simulink model "ProbeModel_Real"  (R2025a)
settings: Solver=ode23tb  StartTime=0.0  StopTime=1000  MaxStep=0.1  RelTol=1e-3
model workspace (MAT data in the model file):
  probe_base_wl = 88.24
  probe_top_wl = 103.68
libraries: simulink x2
settings Model: DataDictionary=FuelGaugingData.sldd  Creator=mkelley  LastModifiedBy=mkelley

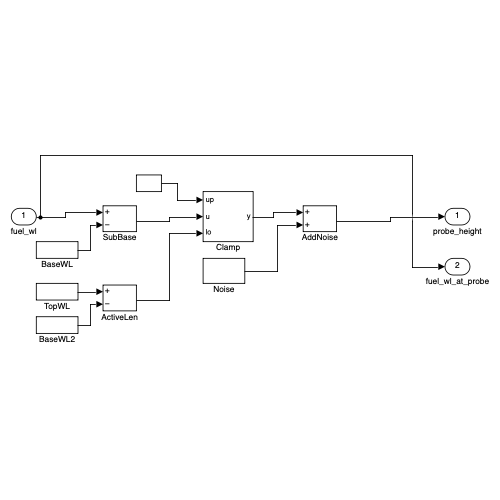
[thumbnail: Simulink's stored preview of the top-level diagram]
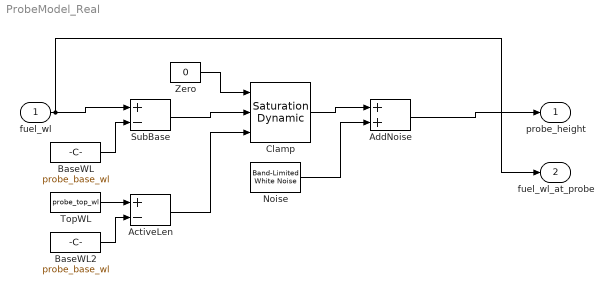
== system ProbeModel_Real ==
  fuel_wl : Inport
  ActiveLen : Sum  Inputs=+-
  AddNoise : Sum
  BaseWL : Constant  Value=probe_base_wl
  BaseWL2 : Constant  Value=probe_base_wl
  Clamp : simulink/Discontinuities/Saturation Dynamic  OutMin=[]  OutMax=[]  OutDataTypeStr=Inherit: Same as second input  OutDataType=fixdt(1, 16)  OutScaling=2^-10  DoSatur=off
  Noise : simulink/Sources/Band-Limited White Noise  Cov=0.0004  Ts=0.1  seed=[23341]
  SubBase : Sum  Inputs=+-
  TopWL : Constant  Value=probe_top_wl
  Zero : Constant  Value=0
  probe_height : Outport
  fuel_wl_at_probe : Outport  Port=2
  wires:
  fuel_wl/1 -> SubBase/1, fuel_wl_at_probe/1
  BaseWL/1 -> SubBase/2
  TopWL/1 -> ActiveLen/1
  BaseWL2/1 -> ActiveLen/2
  Zero/1 -> Clamp/1
  SubBase/1 -> Clamp/2
  ActiveLen/1 -> Clamp/3
  Clamp/1 -> AddNoise/1
  Noise/1 -> AddNoise/2
  AddNoise/1 -> probe_height/1
